simulink model "Current_control"  (R2016b)
settings: Solver=ode45  StartTime=0.0  StopTime=2.0  RelTol=1e-3
libraries: simulink x1
settings Model: Creator=danielesmn  LastModifiedBy=danielesmn

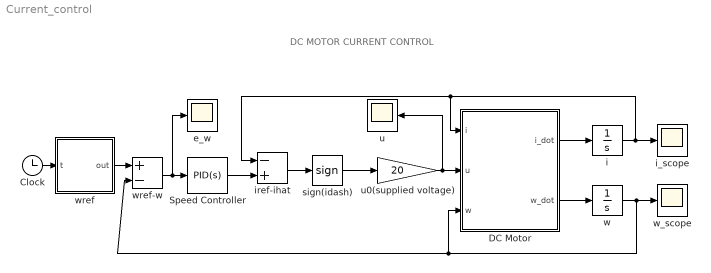
== system Current_control ==
  note: DC MOTOR CURRENT CONTROL
  Clock : Clock
  DC Motor : MATLAB Function  TreatAsAtomicUnit=on
  Speed Controller : simulink/Continuous/PID Controller  Controller=PID  TimeDomain=Continuous-time  SampleTime=-1  IntegratorMethod=Forward Euler  FilterMethod=Forward Euler  Form=Parallel  UseFilter=on  ControllerParametersSource=internal  P=1000  I=100  D=10  N=100  InitialConditionSource=internal  InitialConditionForIntegrator=0  InitialConditionForFilter=0  ExternalReset=none  LimitOutput=off  UpperSaturationLimit=inf  LowerSaturationLimit=-inf  LinearizeAsGain=on  AntiWindupMode=none  Kb=1  TrackingMode=off  Kt=1  PParamMin=[]  PParamMax=[]  IParamMin=[]  IParamMax=[]  DParamMin=[]  DParamMax=[]  NParamMin=[]  NParamMax=[]  KbParamMin=[]  KbParamMax=[]  KtParamMin=[]  KtParamMax=[]  POutMin=[]  POutMax=[]  IOutMin=[]  IOutMax=[]  DOutMin=[]  DOutMax=[]  NOutMin=[]  NOutMax=[]  KbOutMin=[]  KbOutMax=[]  KtOutMin=[]  KtOutMax=[]  IntegratorOutMin=[]  IntegratorOutMax=[]  FilterOutMin=[]  FilterOutMax=[]  SumOutMin=[]  SumOutMax=[]  SumI1OutMin=[]  SumI1OutMax=[]  SumI2OutMin=[]  SumI2OutMax=[]  SumI3OutMin=[]  SumI3OutMax=[]  SumDOutMin=[]  SumDOutMax=[]  SaturationOutMin=[]  SaturationOutMax=[]  IntegratorContinuousStateAttributes=''  IntegratorStateMustResolveToSignalObject=off  IntegratorRTWStateStorageClass=Auto  FilterContinuousStateAttributes=''  FilterStateMustResolveToSignalObject=off  FilterRTWStateStorageClass=Auto  DifferentiatorICPrevScaledInput=0  DifferentiatorOutMin=[]  DifferentiatorOutMax=[]
  e_w : Scope
  i : Integrator
  i_scope : Scope
  iref-ihat : Sum  Inputs=-+
  sign(idash) : Signum  ZeroCross=off
  u : Scope
  u0(supplied voltage) : Gain  Gain=20
  w : Integrator
  w_scope : Scope
  wref : MATLAB Function  TreatAsAtomicUnit=on
  wref-w : Sum  Inputs=+-
  wires:
  DC Motor/1(i_dot) -> i/1
  DC Motor/2(w_dot) -> w/1
  w/1 -> w_scope/1, wref-w/2, DC Motor/3(w)
  Clock/1 -> wref/1(t)
  wref/1(out) -> wref-w/1
  wref-w/1 -> e_w/1, Speed Controller/1
  Speed Controller/1 -> iref-ihat/2
  i/1 -> i_scope/1, iref-ihat/1, DC Motor/1(i)
  iref-ihat/1 -> sign(idash)/1
  sign(idash)/1 -> u0(supplied voltage)/1
  u0(supplied voltage)/1 -> u/1, DC Motor/2(u)

== matlab function Current_control/DC Motor ==
  data: i input; u input; i_dot output; w input; w_dot output
function [i_dot, w_dot] = Dc_Motor(i, u, w) % i: armature current w: shaft speed

%% Model of the DC Motor

L = 0.001;        %Armature inductance (H)
R = 0.5;          %Armature resistance (Ohm)
kt = 0.008;       %Torque constant (Nm/A)
J = 0.001;        %Inertia of the motor rotor (Kg*m^2)
B = 0.01;         %Coefficient of viscous friction (Nm*s/rad)
lambda0 = 0.001;  %Back electromotive force (EMF) constant (V*s/rad)

tauL = B*w;        %Load torque

i_dot = u/L - R/L*i - lambda0/L*w;      %Electrical part model
w_dot = (kt*i - tauL)/J;              %Mechanical part model

== matlab function Current_control/wref ==
  data: t input; out output
function out = input(t)

if t < 0.5 || t>1
    out = -1;
else
    out = 1;
end
